simulink model "G1"  (R2023b)
settings: Solver=VariableStepAuto  StartTime=0.0  StopTime=0.2  RelTol=1e-3
undefined symbols (not defined in the file or in its folder): b, f_final, f_inicial, k, m, t_inicial
settings Model: Creator=klaus  LastModifiedBy=thiag
settings SolverCC: AlgebraicLoopSolver=TrustRegion
settings DebuggingCC: UnconnectedInputMsg=warning  UnconnectedOutputMsg=warning  UnconnectedLineMsg=warning
settings ModelReferenceCC: EnableRefExpFcnMdlSchedulingChecks=on

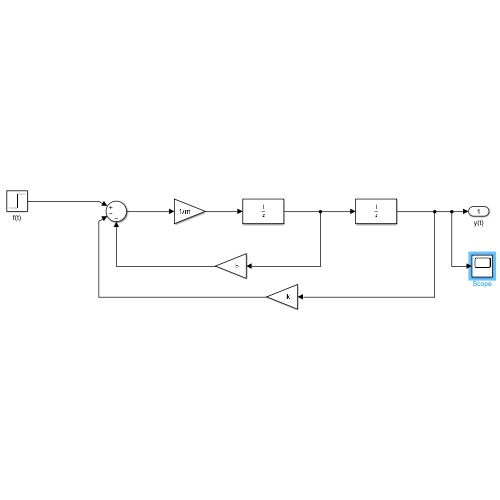
[thumbnail: Simulink's stored preview of the top-level diagram]
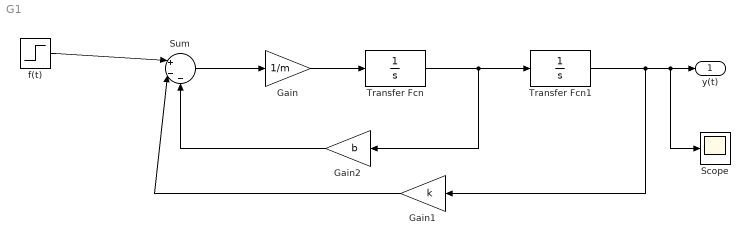
== system G1 ==
  Gain : Gain  Gain=1/m
  Gain1 : Gain  Gain=k
  Gain2 : Gain  Gain=b
  Scope : Scope
  Sum : Sum  Inputs=|+--
  Transfer Fcn : TransferFcn  Denominator=[1 0]
  Transfer Fcn1 : TransferFcn  Denominator=[1 0]
  f(t) : Step  Time=t_inicial  Before=f_inicial  After=f_final  SampleTime=0
  y(t) : Outport
  wires:
  Sum/1 -> Gain/1
  Gain/1 -> Transfer Fcn/1
  Transfer Fcn/1 -> Gain2/1, Transfer Fcn1/1
  Transfer Fcn1/1 -> Gain1/1, Scope/1, y(t)/1
  Gain2/1 -> Sum/3
  Gain1/1 -> Sum/2
  f(t)/1 -> Sum/1
